simulink model "CH06_6"  (R2019a)
settings: Solver=VariableStepAuto  StartTime=0.0  StopTime=10.0  RelTol=1e-3
settings Model: Creator=吳俊逸  LastModifiedBy=吳俊逸

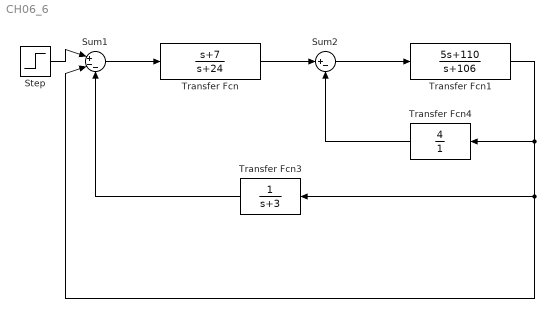
== system CH06_6 ==
  Step : Step  SampleTime=0
  Sum1 : Sum  Inputs=|+--
  Sum2 : Sum  Inputs=|+-
  Transfer Fcn : TransferFcn  Numerator=[1 7]  Denominator=[1 24]
  Transfer Fcn1 : TransferFcn  Numerator=[5 110]  Denominator=[1 106]
  Transfer Fcn3 : TransferFcn  Denominator=[1 3]
  Transfer Fcn4 : TransferFcn  Numerator=[4]  Denominator=[1]
  wires:
  Sum1/1 -> Transfer Fcn/1
  Transfer Fcn3/1 -> Sum1/3
  Step/1 -> Sum1/1
  Transfer Fcn/1 -> Sum2/1
  Sum2/1 -> Transfer Fcn1/1
  Transfer Fcn4/1 -> Sum2/2
  Transfer Fcn1/1 -> Transfer Fcn3/1, Sum1/2, Transfer Fcn4/1
